simulink model "component_6CA185BFF1A8CB94_final_harness"  (R2024b)
settings: Solver=FixedStepDiscrete  StartTime=0.0  StopTime=EV_stop  FixedStep=EV_dt  RelTol=1e-3
libraries: SignalEditorBlockLib x1
settings Model: Creator=menda  LastModifiedBy=menda

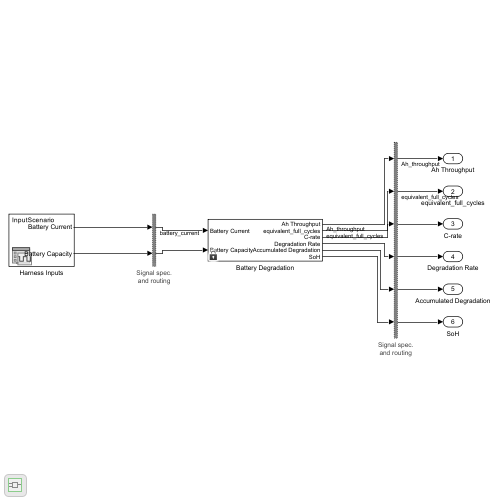
[thumbnail: Simulink's stored preview of the top-level diagram]
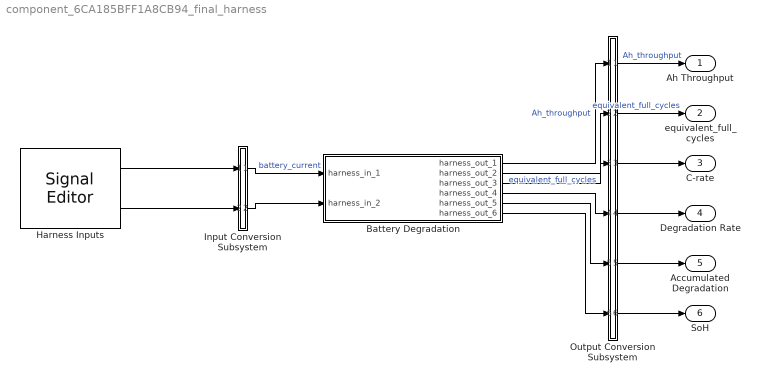
== system component_6CA185BFF1A8CB94_final_harness ==
  Battery Degradation : Subsystem  Tag=__SL_testing_harness_stub_
  Harness Inputs : SignalEditorBlockLib/Signal Editor  FileName=C:\Users\menda\OneDrive\Documentos\HackatonSAE\slprj\mbd_agent\test\EV_Backward_Baseline\component_6CA185BFF1A8CB94_final_harness_HarnessInputs.mat  ActiveScenario=InputScenario  ActiveSignal=Battery Capacity  IsBus=off  OutputBusObjectStr=Bus: BusObject  SampleTime=0  Interpolate=off  ZeroCross=off  OutputAfterFinalValue=Setting to zero  Unit=inherit  PreserveSignalName=on  ApplySigPropsToAllScenarios=on  ApplySigPropsToAllSignals=off
  Input Conversion Subsystem : Subsystem  Tag=__SLT_ICS__  Description=|
      | Signal spec.
      | and routing
      settings: AttributesFormatString=%<Description>
  Output Conversion Subsystem : Subsystem  Tag=__SLT_OCS__  Description=|
      | Signal spec.
      | and routing
      settings: AttributesFormatString=%<Description>
  Ah Throughput : Outport
  equivalent_full_cycles : Outport  Port=2
  C-rate : Outport  Port=3
  Degradation Rate : Outport  Port=4
  Accumulated Degradation : Outport  Port=5
  SoH : Outport  Port=6
  wires:
  Harness Inputs/1 -> Input Conversion Subsystem/1(Inport_1)
  Harness Inputs/2 -> Input Conversion Subsystem/2(Inport_2)
  Output Conversion Subsystem/1(Outport_1) -> Ah Throughput/1  "Ah_throughput"
  Output Conversion Subsystem/2(Outport_2) -> equivalent_full_cycles/1  "equivalent_full_cycles"
  Output Conversion Subsystem/3(Outport_3) -> C-rate/1
  Output Conversion Subsystem/4(Outport_4) -> Degradation Rate/1
  Output Conversion Subsystem/5(Outport_5) -> Accumulated Degradation/1
  Output Conversion Subsystem/6(Outport_6) -> SoH/1
  Input Conversion Subsystem/1(Outport_1) -> Battery Degradation/1(harness_in_1)  "battery_current"
  Input Conversion Subsystem/2(Outport_2) -> Battery Degradation/2(harness_in_2)
  Battery Degradation/1(harness_out_1) -> Output Conversion Subsystem/1(Inport_1)  "Ah_throughput"
  Battery Degradation/2(harness_out_2) -> Output Conversion Subsystem/2(Inport_2)  "equivalent_full_cycles"
  Battery Degradation/3(harness_out_3) -> Output Conversion Subsystem/3(Inport_3)
  Battery Degradation/4(harness_out_4) -> Output Conversion Subsystem/4(Inport_4)
  Battery Degradation/5(harness_out_5) -> Output Conversion Subsystem/5(Inport_5)
  Battery Degradation/6(harness_out_6) -> Output Conversion Subsystem/6(Inport_6)

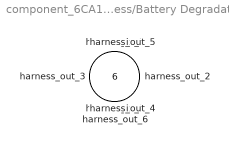
== system component_6CA185BFF1A8CB94_final_harness/Battery Degradation ==
  harness_in_1 : Inport
  harness_in_2 : Inport  Port=2
  harness_out_1 : Outport
  harness_out_2 : Outport  Port=2
  harness_out_3 : Outport  Port=3
  harness_out_4 : Outport  Port=4
  harness_out_5 : Outport  Port=5
  harness_out_6 : Outport  Port=6

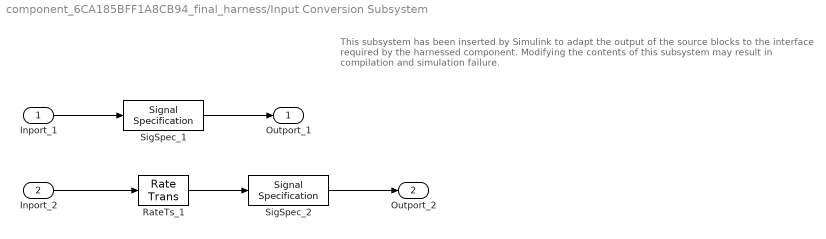
== system component_6CA185BFF1A8CB94_final_harness/Input Conversion Subsystem ==
  note: This subsystem has been inserted by Simulink to adapt the output of the source blocks to the interface required by the harnessed component.
      |  Modifying the contents of this subsystem may result in compilation and simulation failure.
  Inport_1 : Inport
  Inport_2 : Inport  Port=2
  RateTs_1 : RateTransition  OutPortSampleTime=[-1, 0]
  SigSpec_1 : SignalSpecification  OutDataTypeStr=double  Dimensions=[1]  SampleTime=0.1
  SigSpec_2 : SignalSpecification  OutDataTypeStr=double  Dimensions=[1]  SampleTime=[-1, 0]
  Outport_1 : Outport
  Outport_2 : Outport  Port=2
  wires:
  SigSpec_1/1 -> Outport_1/1
  Inport_1/1 -> SigSpec_1/1
  SigSpec_2/1 -> Outport_2/1
  RateTs_1/1 -> SigSpec_2/1
  Inport_2/1 -> RateTs_1/1

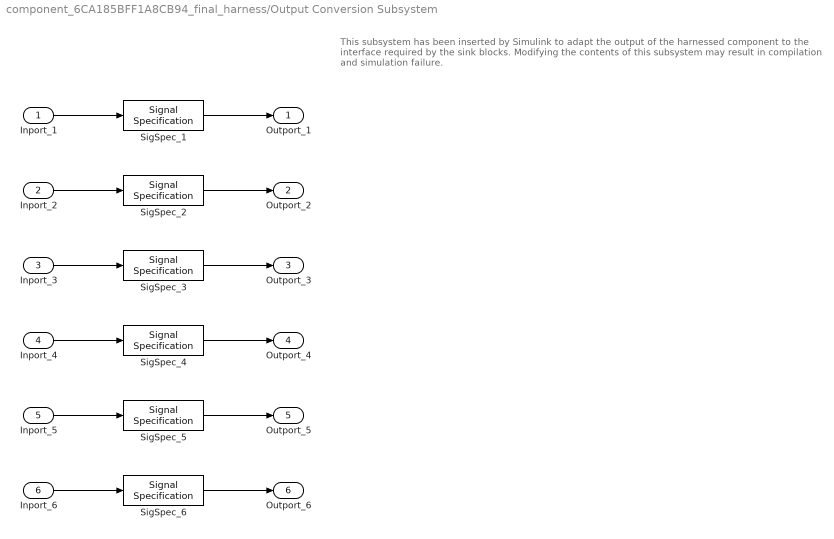
== system component_6CA185BFF1A8CB94_final_harness/Output Conversion Subsystem ==
  note: This subsystem has been inserted by Simulink to adapt the output of the harnessed component to the interface required by the sink blocks.
      |  Modifying the contents of this subsystem may result in compilation and simulation failure.
  Inport_1 : Inport
  Inport_2 : Inport  Port=2
  Inport_3 : Inport  Port=3
  Inport_4 : Inport  Port=4
  Inport_5 : Inport  Port=5
  Inport_6 : Inport  Port=6
  SigSpec_{1..6} (6 alike) : SignalSpecification  OutDataTypeStr=double  Dimensions=[1]  SampleTime=0.1
  Outport_1 : Outport
  Outport_2 : Outport  Port=2
  Outport_3 : Outport  Port=3
  Outport_4 : Outport  Port=4
  Outport_5 : Outport  Port=5
  Outport_6 : Outport  Port=6
  wires:
  Inport_1/1 -> SigSpec_1/1
  SigSpec_1/1 -> Outport_1/1
  Inport_2/1 -> SigSpec_2/1
  SigSpec_2/1 -> Outport_2/1
  Inport_3/1 -> SigSpec_3/1
  SigSpec_3/1 -> Outport_3/1
  Inport_4/1 -> SigSpec_4/1
  SigSpec_4/1 -> Outport_4/1
  Inport_5/1 -> SigSpec_5/1
  SigSpec_5/1 -> Outport_5/1
  Inport_6/1 -> SigSpec_6/1
  SigSpec_6/1 -> Outport_6/1
